simulink model "MotorModelling"  (R2024a)
settings: Solver=VariableStepAuto  StartTime=0.0  StopTime=0.5  RelTol=1e-3
libraries: dspindex x6
settings Model: Creator=User  LastModifiedBy=User

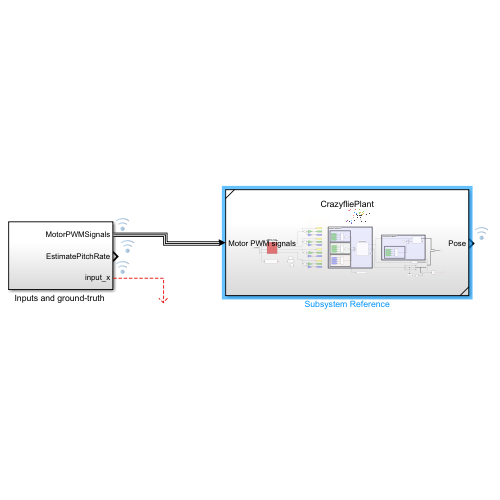
[thumbnail: Simulink's stored preview of the top-level diagram]
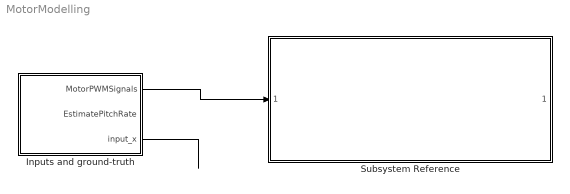
== system MotorModelling ==
  "Inputs and ground-truth " : Subsystem  Tag=Signal Editor
  Subsystem Reference : Subsystem  ReferencedSubsystem=CrazyfliePlant
  wires:
  "Inputs and ground-truth "/1(MotorPWMSignals) -> Subsystem Reference/1
  "Inputs and ground-truth "/3(input_x) -> ?

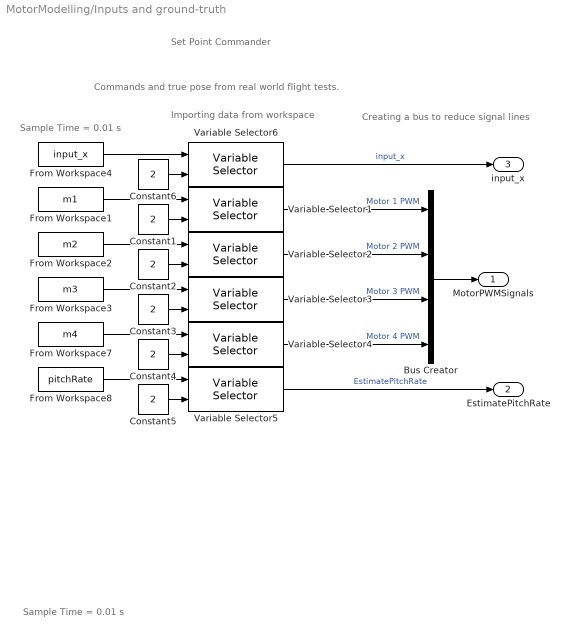
== system MotorModelling/Inputs and ground-truth  ==
  note: Creating a bus to reduce signal lines
  note: Set Point Commander
  note: Importing data from workspace
  note: Commands and true pose from real world flight tests.
  note: Sample Time = 0.01 s
  note: Sample Time = 0.01 s
  Bus Creator : BusCreator  Inputs=4
  Constant{1..6} (6 alike) : Constant  Value=2
  From Workspace1 : FromWorkspace  VariableName=m1  SampleTime=0.01  OutputAfterFinalValue=Setting to zero
  From Workspace2 : FromWorkspace  VariableName=m2  SampleTime=0.01  OutputAfterFinalValue=Setting to zero
  From Workspace3 : FromWorkspace  VariableName=m3  SampleTime=0.01  OutputAfterFinalValue=Setting to zero
  From Workspace4 : FromWorkspace  VariableName=input_x  SampleTime=0.01  OutputAfterFinalValue=Setting to zero
  From Workspace7 : FromWorkspace  VariableName=m4  SampleTime=0.002  OutputAfterFinalValue=Setting to zero
  From Workspace8 : FromWorkspace  VariableName=pitchRate  SampleTime=0.002  OutputAfterFinalValue=Setting to zero
  Variable Selector{1..6} (6 alike) : dspindex/Variable Selector  NumInputs=1  rowsOrCols=Columns  IdxMode=Variable  Elements=[1 3]  ZerOneIdxMode=One-based  errmode=Clip Index  FillMode=off  FillValues=0
  MotorPWMSignals : Outport
  EstimatePitchRate : Outport  Port=2
  input_x : Outport  Port=3
  wires:
  From Workspace1/1 -> Variable Selector1/1
  From Workspace2/1 -> Variable Selector2/1
  From Workspace3/1 -> Variable Selector3/1
  Variable Selector4/1 -> Bus Creator/4  "Motor 4 PWM"
  Variable Selector3/1 -> Bus Creator/3  "Motor 3 PWM"
  Variable Selector2/1 -> Bus Creator/2  "Motor 2 PWM"
  Variable Selector1/1 -> Bus Creator/1  "Motor 1 PWM"
  Constant1/1 -> Variable Selector1/2
  Constant2/1 -> Variable Selector2/2
  Constant3/1 -> Variable Selector3/2
  Constant4/1 -> Variable Selector4/2
  Constant5/1 -> Variable Selector5/2
  From Workspace7/1 -> Variable Selector4/1
  From Workspace8/1 -> Variable Selector5/1
  Variable Selector5/1 -> EstimatePitchRate/1  "EstimatePitchRate"
  Bus Creator/1 -> MotorPWMSignals/1
  Variable Selector6/1 -> input_x/1  "input_x"
  From Workspace4/1 -> Variable Selector6/1
  Constant6/1 -> Variable Selector6/2
